simulink model "robust_tracking_extended_estimator_bonus"  (R2020b)
settings: Solver=ode45  StartTime=0.0  StopTime=5  RelTol=1e-3
undefined symbols (not defined in the file): Aest, Beq_hat, Best, Cest, daq, Dest, drv, gbox, Jeq_hat, K3, mot, rads2rpm, rpm2rads, sens, step_size, tau_hat
settings Model: Creator=utente  LastModifiedBy=giuli
settings DataIOCC: ReturnWorkspaceOutputs=off

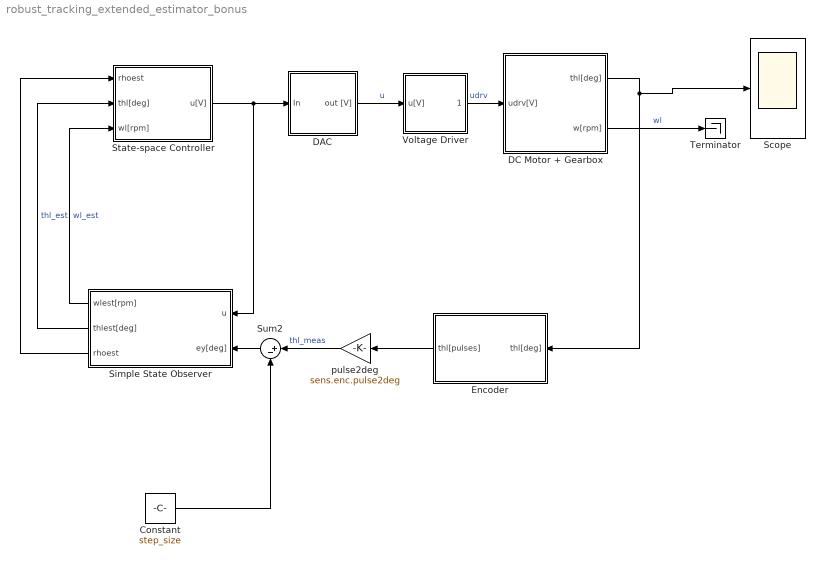
== system robust_tracking_extended_estimator_bonus ==
  Constant : Constant  Value=step_size
  DAC : Subsystem
  DC Motor + Gearbox : Subsystem
  Encoder : Subsystem
  Scope : Scope
  Simple State Observer : Subsystem
  State-space Controller : Subsystem
  Sum2 : Sum  Inputs=|+-
  Terminator : Terminator
  Voltage Driver : Subsystem
  pulse2deg : Gain  Gain=sens.enc.pulse2deg
  wires:
  State-space Controller/1(u[V]) -> Simple State Observer/1(u), DAC/1(In)
  DAC/1(out [V]) -> Voltage Driver/1(u[V])  "u"
  Voltage Driver/1(udrv[V]) -> DC Motor + Gearbox/1(udrv[V])  "udrv"
  Encoder/1(thl[pulses]) -> pulse2deg/1
  DC Motor + Gearbox/1(thl[deg]) -> Scope/1, Encoder/1(thl[deg])
  Sum2/1 -> Simple State Observer/2(ey[deg])
  pulse2deg/1 -> Sum2/1  "thl_meas"
  Simple State Observer/3(rhoest) -> State-space Controller/1(rhoest)
  Simple State Observer/2(thlest[deg]) -> State-space Controller/2(thl[deg])  "thl_est"
  Simple State Observer/1(wlest[rpm]) -> State-space Controller/3(wl[rpm])  "wl_est"
  Constant/1 -> Sum2/2
  DC Motor + Gearbox/2(w[rpm]) -> Terminator/1  "wl"

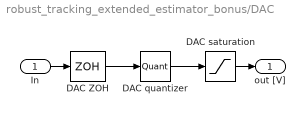
== system robust_tracking_extended_estimator_bonus/DAC ==
  In : Inport
  DAC quantizer : Quantizer  QuantizationInterval=daq.dac.q
  DAC saturation : Saturate  UpperLimit=daq.dac.fs  LowerLimit=-daq.dac.fs
  DAC ZOH : ZeroOrderHold  SampleTime=0.001
  out [V] : Outport
  wires:
  DAC ZOH/1 -> DAC quantizer/1
  DAC quantizer/1 -> DAC saturation/1
  In/1 -> DAC ZOH/1
  DAC saturation/1 -> out [V]/1

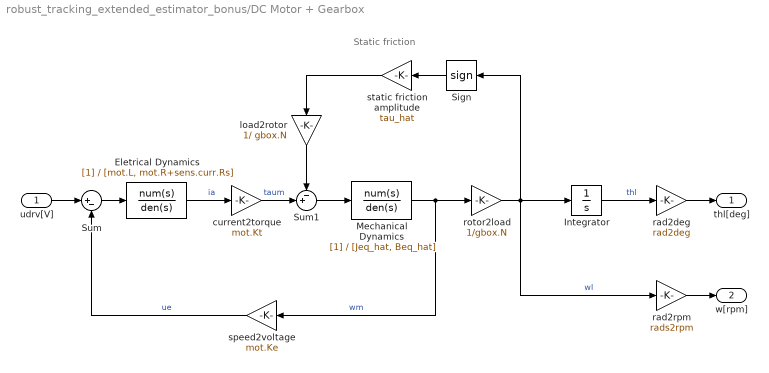
== system robust_tracking_extended_estimator_bonus/DC Motor + Gearbox ==
  note: Static friction
  udrv[V] : Inport
  Eletrical Dynamics : TransferFcn  Denominator=[mot.L, mot.R+sens.curr.Rs]
  Integrator : Integrator
  Mechanical Dynamics : TransferFcn  Denominator=[Jeq_hat, Beq_hat]
  Sign : Signum  ZeroCross=off
  Sum : Sum  Inputs=|+-
  Sum1 : Sum  Inputs=-+|
  current2torque : Gain  Gain=mot.Kt
  load2rotor : Gain  Gain=1/ gbox.N
  rad2deg : Gain  Gain=rad2deg
  "rad2rpm " : Gain  Gain=rads2rpm
  rotor2load : Gain  Gain=1/gbox.N
  speed2voltage : Gain  Gain=mot.Ke
  static friction amplitude : Gain  Gain=tau_hat
  thl[deg] : Outport  VectorParamsAs1DForOutWhenUnconnected=off
  w[rpm] : Outport  Port=2  VectorParamsAs1DForOutWhenUnconnected=off
  wires:
  Eletrical Dynamics/1 -> current2torque/1  "ia"
  udrv[V]/1 -> Sum/1
  Sum/1 -> Eletrical Dynamics/1
  current2torque/1 -> Sum1/2  "taum"
  Sum1/1 -> Mechanical Dynamics/1
  Mechanical Dynamics/1 -> rotor2load/1, speed2voltage/1  "wm"
  rotor2load/1 -> Integrator/1, "rad2rpm "/1, Sign/1  "wl"
  Integrator/1 -> rad2deg/1  "thl"
  rad2deg/1 -> thl[deg]/1
  "rad2rpm "/1 -> w[rpm]/1
  static friction amplitude/1 -> load2rotor/1
  Sign/1 -> static friction amplitude/1
  speed2voltage/1 -> Sum/2  "ue"
  load2rotor/1 -> Sum1/1

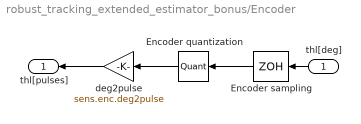
== system robust_tracking_extended_estimator_bonus/Encoder ==
  thl[deg] : Inport
  Encoder quantization : Quantizer  QuantizationInterval=sens.enc.pulse2deg
  Encoder sampling : ZeroOrderHold  SampleTime=-1
  deg2pulse : Gain  Gain=sens.enc.deg2pulse
  thl[pulses] : Outport
  wires:
  thl[deg]/1 -> Encoder sampling/1
  Encoder quantization/1 -> deg2pulse/1
  Encoder sampling/1 -> Encoder quantization/1
  deg2pulse/1 -> thl[pulses]/1

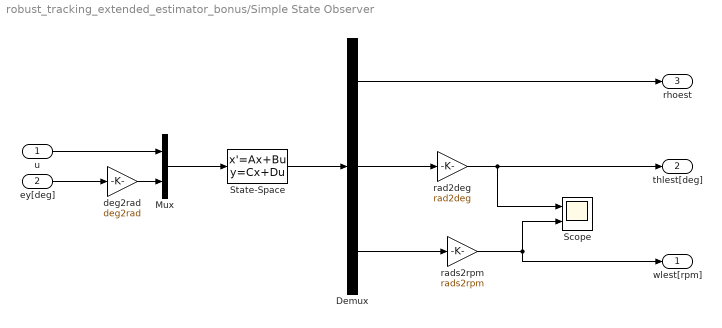
== system robust_tracking_extended_estimator_bonus/Simple State Observer ==
  u : Inport
  ey[deg] : Inport  Port=2
  Demux : Demux  Outputs=3
  Mux : Mux  Inputs=2
  Scope : Scope  NumInputPorts=2
  State-Space : StateSpace  A=Aest  B=Best  C=Cest  D=Dest  InitialCondition=0
  deg2rad : Gain  Gain=deg2rad
  rad2deg : Gain  Gain=rad2deg
  rads2rpm : Gain  Gain=rads2rpm
  wlest[rpm] : Outport
  thlest[deg] : Outport  Port=2
  rhoest : Outport  Port=3
  wires:
  Mux/1 -> State-Space/1
  State-Space/1 -> Demux/1
  ey[deg]/1 -> deg2rad/1
  u/1 -> Mux/1
  rads2rpm/1 -> wlest[rpm]/1, Scope/2
  rad2deg/1 -> thlest[deg]/1, Scope/1
  deg2rad/1 -> Mux/2
  Demux/1 -> rhoest/1
  Demux/2 -> rad2deg/1
  Demux/3 -> rads2rpm/1

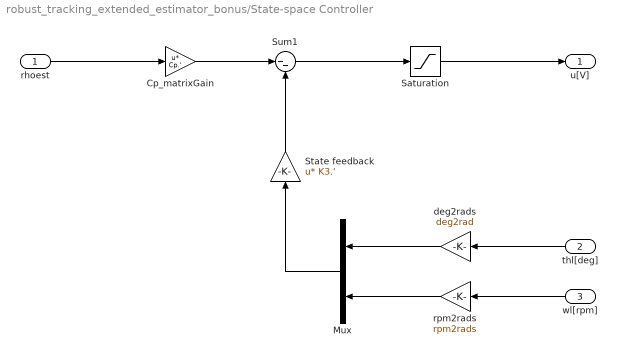
== system robust_tracking_extended_estimator_bonus/State-space Controller ==
  rhoest : Inport
  thl[deg] : Inport  Port=2
  wl[rpm] : Inport  Port=3
  Cp_matrixGain : Gain  Gain=Cp.'  Multiplication=Matrix(u*K)
  Mux : Mux  Inputs=2
  Saturation : Saturate  UpperLimit=10  LowerLimit=-10
  State feedback : Gain  Gain=K3.'  Multiplication=Matrix(u*K)
  Sum1 : Sum  Inputs=|--
  deg2rads : Gain  Gain=deg2rad
  rpm2rads : Gain  Gain=rpm2rads
  u[V] : Outport
  wires:
  Saturation/1 -> u[V]/1
  deg2rads/1 -> Mux/1
  rpm2rads/1 -> Mux/2
  thl[deg]/1 -> deg2rads/1
  wl[rpm]/1 -> rpm2rads/1
  Mux/1 -> State feedback/1
  rhoest/1 -> Cp_matrixGain/1
  State feedback/1 -> Sum1/2
  Cp_matrixGain/1 -> Sum1/1
  Sum1/1 -> Saturation/1

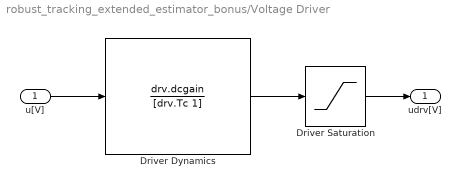
== system robust_tracking_extended_estimator_bonus/Voltage Driver ==
  u[V] : Inport
  Driver Dynamics : TransferFcn  Numerator=drv.dcgain  Denominator=[drv.Tc 1]
  Driver Saturation : Saturate  UpperLimit=12  LowerLimit=-12
  udrv[V] : Outport
  wires:
  Driver Dynamics/1 -> Driver Saturation/1
  Driver Saturation/1 -> udrv[V]/1
  u[V]/1 -> Driver Dynamics/1
